simulink model "Controller_First_Test"  (R2019b)
settings: Solver=VariableStepAuto  StartTime=0.0  StopTime=time  FixedStep=1  RelTol=1e-3
undefined symbols (not defined in the file or in its folder): A, B, C, D, K, K_u, sysKF, T_ambient, T_setpoint1, T_setpoint2
libraries: simulink x4, realtime_pacer_lib x1, cstblocks x1
settings Model: Creator=Presentatie  LastModifiedBy=Presentatie

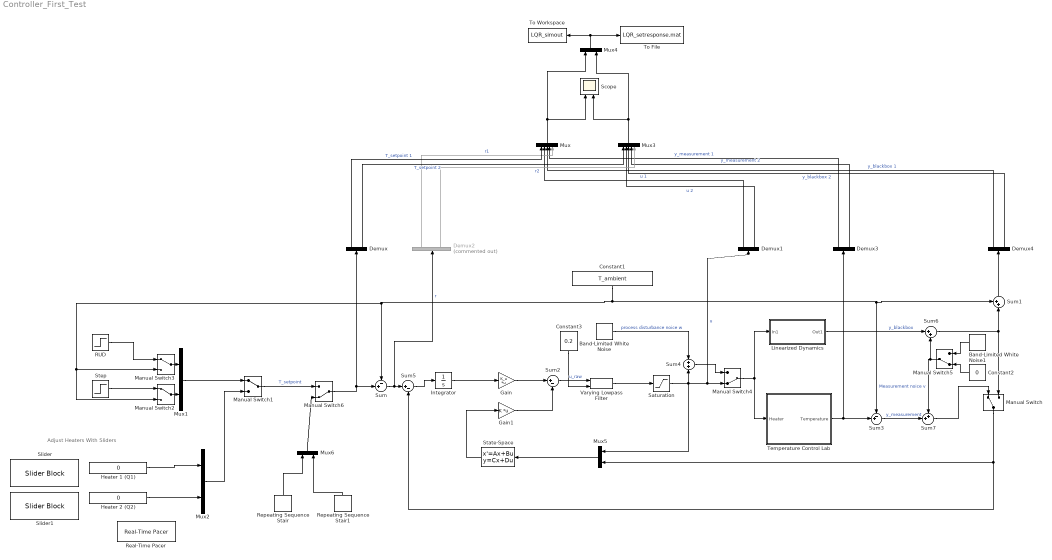
== system Controller_First_Test ==
  note: Adjust Heaters With Sliders
  Band-Limited White Noise : simulink/Sources/Band-Limited White Noise  Cov=[1]  Ts=0.1  seed=[23341]
  Band-Limited White Noise1 : simulink/Sources/Band-Limited White Noise  Cov=[0.1]  Ts=0.1  seed=[23341]
  Constant1 : Constant  Value=T_ambient
  Constant2 : Constant  Value=0
  Constant3 : Constant  Value=0.2
  Demux{,1,3..4} (4 alike) : Demux  Outputs=2
  Demux2 : Demux  Commented=on  Outputs=2
  Gain : Gain  Gain=K_u  Multiplication=Matrix(K*u)
  Gain1 : Gain  Gain=K  Multiplication=Matrix(K*u)
  Heater 1 (Q1) : Constant  Value=0
  Heater 2 (Q2) : Constant  Value=0
  Integrator : Integrator  InitialCondition=[-5 -5]  LimitOutput=on  UpperSaturationLimit=2E3  LowerSaturationLimit=-2E3
  Linearized Dynamics : Subsystem
  Manual Switch{,1..3} (4 alike) : ManualSwitch
  Manual Switch4 : ManualSwitch  CurrentSetting=0
  Manual Switch5 : ManualSwitch  CurrentSetting=0
  Manual Switch6 : ManualSwitch  CurrentSetting=0
  Mux : Mux  Inputs=5
  Mux{1..2,4..6} (5 alike) : Mux  Inputs=2
  Mux3 : Mux  Inputs=5
  "RUD " : Step  Time=30  Before=25  After=35  SampleTime=0
  Real-Time Pacer : realtime_pacer_lib/Real-Time Pacer  simTimePerRealTime=1
  Repeating Sequence Stair : simulink/Sources/Repeating Sequence Stair  OutValues=T_setpoint1'  tsamp=1  OutMin=[]  OutMax=[]  OutDataTypeStr=double  OutputDataTypeScalingMode=double  OutDataType=fixdt(0,8)  ConRadixGroup=Best Precision: Vector-wise  OutScaling=2^-12
  Repeating Sequence Stair1 : simulink/Sources/Repeating Sequence Stair  OutValues=T_setpoint2'  tsamp=1  OutMin=[]  OutMax=[]  OutDataTypeStr=double  OutputDataTypeScalingMode=double  OutDataType=fixdt(0,8)  ConRadixGroup=Best Precision: Vector-wise  OutScaling=2^-12
  Saturation : Saturate  UpperLimit=100  LowerLimit=0
  Scope : Scope  NumInputPorts=2
  Slider : SliderBlock  TickInterval=20
  Slider1 : SliderBlock  TickInterval=20
  State-Space : StateSpace  A=sysKF.a  B=sysKF.b  C=sysKF.c  D=sysKF.d  InitialCondition=[0 0 5 5]
  Step : Step  Time=60  Before=25  After=35  SampleTime=0
  Sum : Sum  Inputs=-+|
  Sum1 : Sum  Inputs=++|
  Sum2 : Sum  Inputs=|+-
  Sum3 : Sum  Inputs=-+|
  Sum4 : Sum  Inputs=+|+
  Sum5 : Sum  Inputs=|+-
  Sum6 : Sum  Inputs=|++
  Sum7 : Sum  Inputs=++|
  Temperature Control Lab : Subsystem
      mask Display: image('tclab.png');
  To File : ToFile  Filename=LQR_setresponse.mat  SaveFormat=Timeseries
  To Workspace : ToWorkspace  VariableName=LQR_simout  SaveFormat=Timeseries  SampleTime=-1
  Varying Lowpass Filter : cstblocks/Linear Parameter Varying/Varying Lowpass Filter  N=1
      settings: SourceProductName=Control System Toolbox
  wires:
  Mux/1 -> Scope/1, Mux4/1
  Heater 2 (Q2)/1 -> Mux2/2
  Mux2/1 -> Manual Switch1/2
  Heater 1 (Q1)/1 -> Mux2/1
  Gain/1 -> Sum2/1
  Gain1/1 -> Sum2/2
  Temperature Control Lab/1(Temperature) -> Demux3/1, Sum3/2
  Saturation/1 -> Mux5/1, Sum4/2, Manual Switch4/2, Demux1/1  "u"
  Sum/1 -> Demux2/1, Sum5/1  "r"
  Sum5/1 -> Integrator/1
  Demux1/1 -> Mux/2  "u 1"
  Demux4/1 -> Mux/3  "y_blackbox 1"
  Demux3/1 -> Mux/4  "y_measurement 1"
  Demux1/2 -> Mux3/2  "u 2"
  Demux4/2 -> Mux3/3  "y_blackbox 2"
  Demux3/2 -> Mux3/4  "y_measurement 2"
  Mux3/1 -> Scope/2, Mux4/2
  Mux4/1 -> To Workspace/1, To File/1
  Constant3/1 -> Varying Lowpass Filter/2
  Sum2/1 -> Varying Lowpass Filter/1  "u_raw"
  Integrator/1 -> Gain/1
  Demux2/1 -> Mux/5  "r1"
  Demux2/2 -> Mux3/5  "r2"
  Demux/1 -> Mux/1  "T_setpoint 1"
  Demux/2 -> Mux3/1  "T_setpoint 2"
  Mux1/1 -> Manual Switch1/1
  Constant1/1 -> Sum1/1, Sum3/1, Manual Switch2/2, Manual Switch3/2, Sum/1
  Step/1 -> Manual Switch2/1
  Manual Switch2/1 -> Mux1/2
  Manual Switch3/1 -> Mux1/1
  "RUD "/1 -> Manual Switch3/1
  Sum1/1 -> Demux4/1
  Manual Switch/1 -> Sum5/2, Mux5/2
  Band-Limited White Noise/1 -> Sum4/1  "process disturbance noice w"
  Manual Switch4/1 -> Temperature Control Lab/1(Heater), Linearized Dynamics/1(In1)
  Sum4/1 -> Manual Switch4/1
  Linearized Dynamics/1(Out1) -> Sum6/1  "y_blackbox"
  Sum6/1 -> Sum1/2, Manual Switch/2
  Sum3/1 -> Sum7/2  "y_measurement"
  Sum7/1 -> Manual Switch/1
  Constant2/1 -> Manual Switch5/2
  Band-Limited White Noise1/1 -> Manual Switch5/1
  Manual Switch5/1 -> Sum6/2, Sum7/1  "Measurement noice v"
  Mux5/1 -> State-Space/1
  Varying Lowpass Filter/1 -> Saturation/1
  State-Space/1 -> Gain1/1
  Manual Switch6/1 -> Demux/1, Sum/2
  Manual Switch1/1 -> Manual Switch6/1  "T_setpoint"
  Repeating Sequence Stair1/1 -> Mux6/2
  Repeating Sequence Stair/1 -> Mux6/1
  Mux6/1 -> Manual Switch6/2

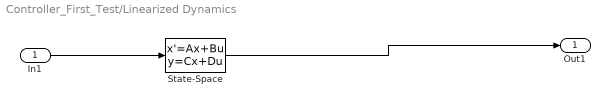
== system Controller_First_Test/Linearized Dynamics ==
  In1 : Inport
  State-Space : StateSpace  A=A  B=B  C=C  D=D  InitialCondition=0
  Out1 : Outport
  wires:
  In1/1 -> State-Space/1
  State-Space/1 -> Out1/1

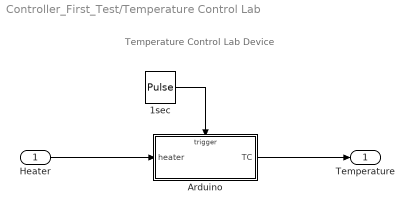
== system Controller_First_Test/Temperature Control Lab ==
  note: Temperature Control Lab Device
  Heater : Inport
  1sec : DiscretePulseGenerator  PulseType=Time based  Period=1  PulseWidth=50
  Arduino : Subsystem  TreatAsAtomicUnit=on
  Temperature : Outport  VectorParamsAs1DForOutWhenUnconnected=off
  wires:
  1sec/1 -> Arduino/Trigger
  Arduino/1(TC) -> Temperature/1
  Heater/1 -> Arduino/1(heater)

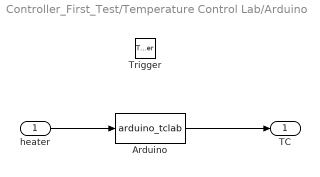
== system Controller_First_Test/Temperature Control Lab/Arduino ==
  heater : Inport  LatchByDelayingOutsideSignal=on
  Trigger : TriggerPort  VariantControl=Variant
  Arduino : MATLABFcn  MATLABFcn=arduino_tclab
  TC : Outport  InitialOutput=[23 23]  VectorParamsAs1DForOutWhenUnconnected=off
  wires:
  heater/1 -> Arduino/1
  Arduino/1 -> TC/1
